simulink model "operativobuono"  (R2024a)
settings: Solver=VariableStepAuto  StartTime=0.0  StopTime=70  RelTol=1e-3
undefined symbols (not defined in the file or in its folder): DiscIntNeverNeededParam
settings Model: Creator=ThinkPad  LastModifiedBy=UTENTE
settings ModelReferenceCC: EnableRefExpFcnMdlSchedulingChecks=on
settings RTWCC: GPUComputeCapability=3.5

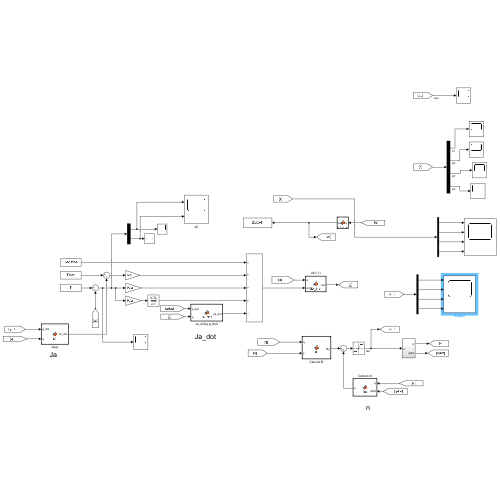
[thumbnail: Simulink's stored preview of the top-level diagram]
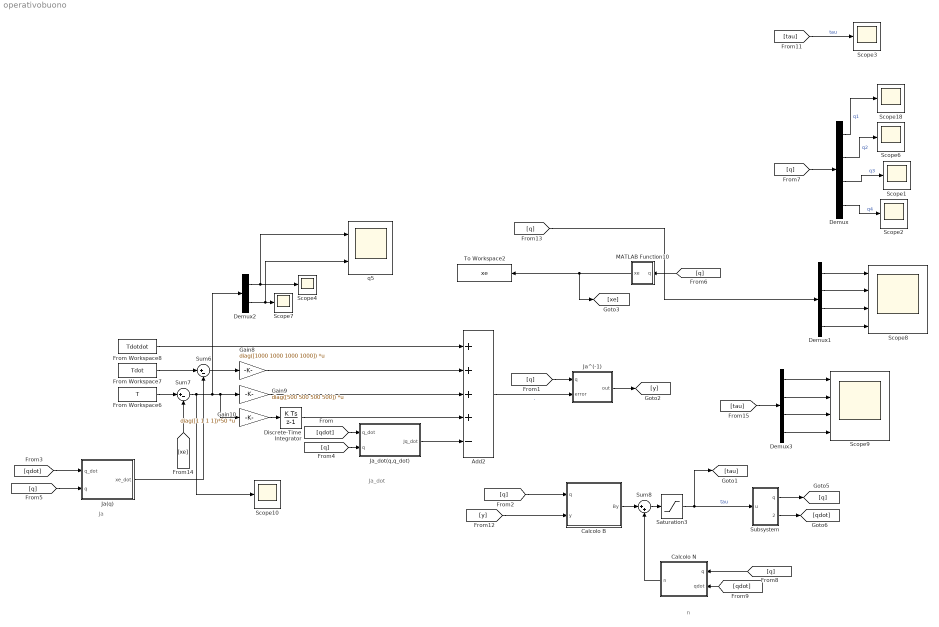
== system operativobuono ==
  note: n
  note: Ja
  note: Ja_dot
  Add2 : Sum  Inputs=++++-
  Calcolo B : MATLAB Function  TreatAsAtomicUnit=on
  Calcolo N : MATLAB Function  TreatAsAtomicUnit=on
  Demux : Demux
  Demux1 : Demux
  Demux2 : Demux  Outputs=[3 1]
  Demux3 : Demux
  Discrete-Time Integrator : DiscreteIntegrator  InitialCondition=[0 0 0 0]'  SampleTime=0.001  ICPrevOutput=DiscIntNeverNeededParam  ICPrevScaledInput=DiscIntNeverNeededParam
  From Workspace6 : FromWorkspace  VariableName=T  SampleTime=0.001
  From Workspace7 : FromWorkspace  VariableName=Tdot  SampleTime=0.001
  From Workspace8 : FromWorkspace  VariableName=Tdotdot
  Gain10 : Gain  Gain=diag([1 1 1 1])*50  Multiplication=Matrix(K*u)
  Gain8 : Gain  Gain=diag([1000 1000 1000 1000])  Multiplication=Matrix(K*u)
  Gain9 : Gain  Gain=diag([500 500 500 500])  Multiplication=Matrix(K*u)
  Ja(q) : MATLAB Function  TreatAsAtomicUnit=on
  Ja^(-1) : MATLAB Function  TreatAsAtomicUnit=on
  Ja_dot(q,q_dot) : MATLAB Function  TreatAsAtomicUnit=on
  MATLAB Function10 : MATLAB Function  TreatAsAtomicUnit=on
  Saturation3 : Saturate  UpperLimit=[1 1 1 1]*300  LowerLimit=-[1 1 1 1]*300
  Scope{1..4,6..7,10,18} (8 alike) : Scope
  Scope8 : Scope  NumInputPorts=4
  Scope9 : Scope  NumInputPorts=4
  Subsystem : Subsystem
  Sum6 : Sum  Inputs=|+-
  Sum7 : Sum  Inputs=|+-
  Sum8 : Sum  Inputs=|++
  To Workspace2 : ToWorkspace  VariableName=xe  SampleTime=0.001
  q5 : Scope  NumInputPorts=2
  wires:
  Ja(q)/1(xe_dot) -> Sum6/2
  Demux3/3 -> Scope9/3
  [q] -> MATLAB Function10/1(q)
  Calcolo N/1(n) -> Sum8/2
  [q] -> Demux/1
  Demux3/4 -> Scope9/4
  Gain9/1 -> Add2/3
  [qdot] -> Calcolo N/2(qdot)
  From Workspace8/1 -> Add2/1
  Demux1/2 -> Scope8/2
  Discrete-Time Integrator/1 -> Add2/4
  Demux1/4 -> Scope8/4
  Demux2/1 -> q5/1, Scope4/1
  Demux2/2 -> q5/2, Scope7/1
  Sum7/1 -> Scope10/1, Demux2/1, Gain9/1, Gain10/1
  [y] -> Calcolo B/2(y)
  [q] -> Ja(q)/2(q)
  Demux3/1 -> Scope9/1
  Sum6/1 -> Gain8/1
  Subsystem/1(q) -> [q]
  Sum8/1 -> Saturation3/1
  From Workspace7/1 -> Sum6/1
  From Workspace6/1 -> Sum7/1
  MATLAB Function10/1(xe) -> [xe], To Workspace2/1
  Add2/1 -> Ja^(-1)/2(error)  "."
  Gain10/1 -> Discrete-Time Integrator/1
  [qdot] -> Ja_dot(q,q_dot)/1(q_dot)
  Demux1/3 -> Scope8/3
  Demux1/1 -> Scope8/1
  Calcolo B/1(By) -> Sum8/1
  [q] -> Calcolo N/1(q)
  [q] -> Calcolo B/1(q)
  Gain8/1 -> Add2/2
  [tau] -> Scope3/1  "tau"
  Ja_dot(q,q_dot)/1(Jq_dot) -> Add2/5
  Demux/4 -> Scope2/1  "q4"
  [qdot] -> Ja(q)/1(q_dot)
  Demux3/2 -> Scope9/2
  [q] -> Ja_dot(q,q_dot)/2(q)
  Subsystem/2(qdot) -> [qdot]
  Saturation3/1 -> Subsystem/1(u), [tau]  "tau"
  Demux/2 -> Scope6/1  "q2"
  Ja^(-1)/1(out) -> [y]
  Demux/1 -> Scope18/1  "q1"
  [q] -> Ja^(-1)/1(q)
  Demux/3 -> Scope1/1  "q3"
  [q] -> Demux1/1
  [xe] -> Sum7/2
  [tau] -> Demux3/1

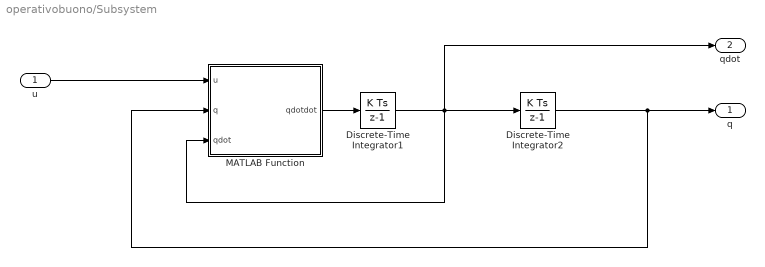
== system operativobuono/Subsystem ==
  u : Inport
  Discrete-Time Integrator1 : DiscreteIntegrator  InitialCondition=[0 0 0 0]'  SampleTime=0.001  ICPrevOutput=DiscIntNeverNeededParam  ICPrevScaledInput=DiscIntNeverNeededParam
  Discrete-Time Integrator2 : DiscreteIntegrator  InitialCondition=[pi/4,pi/6,pi/5,0.5]'  SampleTime=0.001  ICPrevOutput=DiscIntNeverNeededParam  ICPrevScaledInput=DiscIntNeverNeededParam
  MATLAB Function : MATLAB Function  TreatAsAtomicUnit=on
  q : Outport
  qdot : Outport  Port=2
  wires:
  MATLAB Function/1(qdotdot) -> Discrete-Time Integrator1/1
  Discrete-Time Integrator2/1 -> q/1, MATLAB Function/2(q)
  u/1 -> MATLAB Function/1(u)
  Discrete-Time Integrator1/1 -> qdot/1, MATLAB Function/3(qdot), Discrete-Time Integrator2/1

== matlab function operativobuono/Ja(q) ==
  data: q_dot input; q input; xe_dot output
function xe_dot = JA(q_dot, q)

J=[-0.5*sin(q(1))-0.5*sin(q(1)+q(2)) -0.5*sin(q(1)+q(2)) 0 0;
    0.5*cos(q(1))+0.5*cos(q(1)+q(2)) 0.5*cos(q(1)+q(2)) 0 0;
    0 0 -1 0;
    1 1 0 -1];
xe_dot=J*q_dot;
end

== matlab function operativobuono/Ja^(-1) ==
  data: q input; out output; error input
function out= JA_inv(q,error)

J=[-0.5*sin(q(1))-0.5*sin(q(1)+q(2)) -0.5*sin(q(1)+q(2)) 0 0;
    0.5*cos(q(1))+0.5*cos(q(1)+q(2)) 0.5*cos(q(1)+q(2)) 0 0;
    0 0 -1 0;
    1 1 0 -1];

J_inv=inv(J);

 inverse_Jacobian=J_inv;
 out = inverse_Jacobian*error;
end

== matlab function operativobuono/MATLAB Function10 ==
  data: q input; xe output
function xe = cinematica_diretta(q)
% T_4_0=[cos(q(4))*(cos(q(1))*cos(q(2))-sin(q1)*sin(q2))+sin(q(4))*(cos(q1)*sin(q(2))+cos(q(2))*sin(q(1)))   cos(q(4))*(cos(q(1))*sin(q(2))+cos(q(2))*sin(q(1)))-sin(q(4))*(cos(q(1))*cos(q(2))-sin(q(1))*sin(q(2)))  0 cos(q(1))/2+(cos(q(1))*cos(q(2)))/2-(sin(q(1))*sin(q(2)))/2;
%         cos(q(4))*(cos(q(1))*sin(q(2))+cos(q(2))*sin(q(1)))-sin(q(4))*(cos(q(1))*cos(q(2))-sin(q(1))*sin(q(2))) -cos(q(4))*(cos(q(1))*cos(q(2))-sin(q(1))*sin(q(2)))-sin(q(4))*(cos(q(1))*sin(q(2))+cos(q(2))*sin(q(1)))  0 sin(q(1))/2+(cos(q(1))*sin(q(2)))/2+(cos(q(2))*sin(q(2)))/2;
%                       0                                                      0                    -1                                                1-q(3);
%         0                                       0                                         0                                                                                                                                      1];

x_e=[0.5*cos(q(1))+0.5*cos(q(1)+q(2));
    0.5*sin(q(1))+0.5*sin(q(1)+q(2));
        1-q(3);
        q(1)+q(2)-q(4)];
xe=x_e;
end

== matlab function operativobuono/Calcolo N ==
  data: n output; q input; qdot input
function n = fcn(q, qdot)
d0=1;
a1=0.5;
a2=0.5;
l1=0.25;
l2=0.25;
ml1=20;
ml2=20;
ml3=10;
Il1=4;
Il2=4;
Il4=1;
kr1=1;
kr2=1;
kr3=50;
kr4=20;
Im1=0,01;
Im2=0,01;
Im3=0,005;
Im4=0,001;
Fm1=0.00005;
Fm2=0.00005;
Fm3=0.01;
Fm4=0.005;
ml=3;
mm1=0;
mm2=0;
mm3=0;
mm4=0;

Jp_l1=[-l1*sin(q(1)) 0 0  0;
        l1*cos(q(1)) 0 0  0;
        0            0 0  0];
    
Jo_l1=[0 0 0 0;
       0 0 0 0;
       1 0 0 0];
   
Jp_l2=[-a1*sin(q(1))-l2*sin(q(1)+q(2)) -l2*sin(q(1)+q(2)) 0  0;
        a1*cos(q(1))+l2*cos(q(1)+q(2)) +l2*cos(q(1)+q(2)) 0  0;
        0                                      0          0  0];
   
Jo_l2=[0 0 0 0;
       0 0 0 0;
       1 1 0 0];

Jp_l3=[-a1*sin(q(1))-a2*sin(q(1)+q(2)) -a2*sin(q(1)+q(2))  0   0;
        a1*cos(q(1))+a2*cos(q(1)+q(2)) +a2*cos(q(1)+q(2))  0   0;
        0                                               0  -1  0];
Jo_l3=[0 0 0 0;
       0 0 0 0;
       1 1 0 0];
 
Jp_l4=[-a1*sin(q(1))-a2*sin(q(1)+q(2)) -a2*sin(q(1)+q(2))  0   0;
        a1*cos(q(1))+a2*cos(q(1)+q(2)) +a2*cos(q(1)+q(2))  0   0;
        0                                               0  -1  0];
Jo_l4=[0 0 0 0;
       0 0 0 0;
       1 1 0 -1];

Jp_m1=[0 0 0 0;
       0 0 0 0;
       0 0 0 0];
   
Jo_m1=[0 0 0 0;
       0 0 0 0;
       kr1 0 0 0];

Jp_m2=[-a1*sin(q(1)) 0 0 0;
       a1*cos(q(1)) 0 0 0;
           0        0 0 0];
       
Jo_m2=[0 0 0 0;
       0 0 0 0;
       1 kr2 0 0];

Jp_m3=[-a1*sin(q(1))-a2*sin(q(1)+q(2)) -a2*sin(q(1)+q(2))  0 0;
        a1*cos(q(1))+a2*cos(q(1)+q(2)) +a2*cos(q(1)+q(2))  0 0;
                      0                         0          0 0];

Jo_m3=[0 0 0 0;
       0 0 0 0;
       1 1 -kr3 0];

Jp_m4=[-a1*sin(q(1))-a2*sin(q(1)+q(2)) -a2*sin(q(1)+q(2))  0 0;
        a1*cos(q(1))+a2*cos(q(1)+q(2)) +a2*cos(q(1)+q(2))  0 0;
                      0                         0          -1 0];
Jo_m4=[0 0 0 0;
       0 0 0 0;
       1 1 0 -kr4];


Fv=diag([kr1^2*Fm1 kr2^2*Fm2 kr3^2*Fm3 kr4^2*Fm4]);
% Fv=[Fm1 0   0   0;
%     0   Fm2 0   0;
%     0   0   Fm3 0;
%     0   0   0   Fm4];

g=[0 0 -9.81*(ml3) 0]';

Jpl1_dq1=[-l1*cos(q(1)) 0 0 0;
    -l1*sin(q(1)) 0 0 0;
    0 0 0 0];

Jpl2_dq1=[-a1*cos(q(1))-l2*cos(q(1)+q(2)) -l2*cos(q(1)+q(2)) 0 0;
    -a1*sin(q(1))-l2*sin(q(1)+q(2)) -l2*sin(q(1)+q(2)) 0 0;
    0 0 0 0];

Jpl2_dq2=[-a2*cos(q(1)+q(2)) -a2*cos(q(1)+q(2)) 0 0;
    -a2*sin(q(1)+q(2)) -a2*sin(q(1)+q(2)) 0 0;
    0 0 0 0];

Jpl4_dq1=[-a1*cos(q(1))-a2*cos(q(1)+q(2)) -a2*cos(q(1)+q(2)) 0 0;
    -a1*sin(q(1))-a2*sin(q(1)+q(2)) -a2*sin(q(1)+q(2)) 0 0;
    0 0 0 0];

Jpl4_dq2=[-a2*sin(q(1)+q(2)) -a2*sin(q(1)+q(2)) 0 0;
    -a2*cos(q(1)+q(2)) -a2*cos(q(1)+q(2)) 0 0;
    0 0 0 0];

dBdq1=ml1*(Jpl1_dq1'*Jp_l1+Jp_l1'*Jpl1_dq1)+ml2*(Jpl2_dq1'*Jp_l2+Jp_l2'*Jpl2_dq1)...
    +ml3*(Jpl4_dq1'*Jp_l4+Jp_l4'*Jpl4_dq1);

dBdq2=ml2*(Jpl2_dq2'*Jp_l2+Jp_l2'*Jpl2_dq2)+ml3*(Jpl4_dq2'*Jp_l4+Jp_l4'*Jpl4_dq2);

H=zeros(4,4,4);


for i=1:4
    for j=1:4
        for k=1:4
            H(i,j,k)=0;
        end
    end
end

H(1,1,2)=1/2*(dBdq2(1,1)+dBdq1(1,2)-dBdq1(1,2));
H(1,2,1)=H(1,1,2); 
H(1,2,2)=1/2*(dBdq2(1,2)+dBdq2(1,2)-dBdq1(2,2));
H(2,1,1)=1/2*(dBdq1(2,1)+dBdq1(2,1)-dBdq2(1,1));
H(2,1,2)=1/2*(dBdq2(2,1)+dBdq1(2,2)-dBdq2(1,2));
H(2,2,1)=H(2,1,2);
H(2,2,2)=1/2*(dBdq2(2,2)+dBdq2(2,2)-dBdq2(2,2));

C=zeros(4,4);
for i=1:4
    for j=1:4
        C(i,j)=0;
    end
end

for i=1:4
    for j=1:4
        for k=1:4
            r=H(i,j,k)*qdot(k);
            C(i,j)=C(i,j)+r;
        end
    end
end

n=C*qdot+Fv*qdot+g;

end

== matlab function operativobuono/Ja_dot(q,q_dot) ==
  data: q_dot input; q input; Jq_dot output
function Jq_dot = JA_dot(q_dot, q)
J_dot=[-0.5*cos(q(1))*q_dot(1)-0.5*cos(q(1)+q(2))*(q_dot(1)+q_dot(2)) -0.5*cos(q(1)+q(2))*(q_dot(1)+q_dot(2)) 0 0;
    -0.5*sin(q(1))*q_dot(1)-0.5*sin(q(1)+q(2))*(q_dot(1)+q_dot(2)) -0.5*sin(q(1)+q(2))*(q_dot(1)+q_dot(2)) 0 0;
    0 0 0 0;
    0 0 0 0];
Jq_dot=J_dot*q_dot;
end

== matlab function operativobuono/Calcolo B ==
  data: q input; y input; By output
function By = B(q, y)
    d0=1; 
    a1=0.5; 
    a2=0.5; 
    l1=0.25; 
    l2=0.25; 
    ml1=20; 
    ml2=20; 
    ml3=10; 
    ml4=0; 
    Il1=4; 
    Il2=4; 
    Il3=0;
    Il4=1; 
    Kr1=1;
    Kr2=1;
    Kr3=50; 
    Kr4 =20;
    Im1=0.01; 
    Im2=0.01; 
    Im3=0.005; 
    Im4=0.001;
    Fm1=0.00005; 
    Fm2=0.00005; 
    Fm3=0.01; 
    Fm4 =0.005; 
    mm1=0;
    mm2=0;
    mm3=0;
    mm4=0;
    ml=3;
    
    Jp_l1=[-l1*sin(q(1)) 0 0 0; 
            l1*cos(q(1)) 0 0 0; 
            0 0 0 0];
    Jo_l1=[zeros(2,4)
           1 0 0 0];
    
    Jp_l2=[-a1*sin(q(1))-l2*sin(q(1)+q(2)) -l2*sin(q(1)+q(2)) 0 0; 
            a1*cos(q(1))+l2*cos(q(1)+q(2)) l2*cos(q(1)+q(2)) 0 0;
            0 0 0 0];
    Jo_l2=[zeros(2,4)
           1 1 0 0];
    
    Jp_l3=[-a1*sin(q(1))-a2*sin(q(1)+q(2)) -a2*sin(q(1)+q(2)) 0 0; 
            a1*cos(q(1))+a2*cos(q(1)+q(2)) a2*cos(q(1)+q(2)) 0 0;
            0 0 -1 0];
    Jo_l3 = [zeros(2,4)
             1 1 0 0];
    
    Jp_l4=Jp_l3;
    Jo_l4 = [zeros(2,4)
             1 1 0 -1];
    
    Jp_m1 = [0 0 0 0;
             0 0 0 0;
             0 0 0 0];
    Jo_m1 = [zeros(2,4)
             Kr1 0 0 0];
    
    Jp_m2 = [-a1*sin(q(1)) 0 0 0; 
            a1*cos(q(1)) 0 0 0; 
            0 0 0 0];
    Jo_m2 = [zeros(2,4)
             1 Kr2 0 0];
    
    Jp_m3 = [-a1*sin(q(1))-a2*sin(q(1)+q(2)) -a2*sin(q(1)+q(2)) 0 0; 
              a1*cos(q(1))+a2*cos(q(1)+q(2)) a2*cos(q(1)+q(2)) 0 0;
              0 0 0 0];
    Jo_m3 = [zeros(2,4)
             1 1 -Kr3 0];
    
    Jp_m4 = [-a1*sin(q(1))-a2*sin(q(1)+q(2)) -a2*sin(q(1)+q(2)) 0 0; 
              a1*cos(q(1))+a2*cos(q(1)+q(2)) a2*cos(q(1)+q(2)) 0 0;
              0 0 -1 0];
    Jo_m4 = [zeros(2,4)
             1 1 0 -Kr4];
    B1 = ml1*Jp_l1'*Jp_l1+Jo_l1'*Il1*Jo_l1+mm1*Jp_m1'*Jp_m1+Jo_m1'*Im1*Jo_m1;
    B2 = ml2*Jp_l2'*Jp_l2+Jo_l2'*Il2*Jo_l2+mm2*Jp_m2'*Jp_m2+Jo_m2'*Im2*Jo_m2;
    B3 = ml3*Jp_l3'*Jp_l3+Jo_l3'*Il3*Jo_l3+mm3*Jp_m3'*Jp_m3+Jo_m3'*Im3*Jo_m3;
    B4 = (ml4)*Jp_l4'*Jp_l4+Jo_l4'*Il4*Jo_l4+mm4*Jp_m4'*Jp_m4+Jo_m4'*Im4*Jo_m4;
    B = B1+B2+B3+B4;
    
    By=B*y;

end

== matlab function operativobuono/Subsystem/MATLAB Function ==
  data: u input; q input; qdot input; qdotdot output
function qdotdot = fcn(u, q, qdot)
    d0=1; %m
    a1=0.5; %m
    a2=0.5; %m
    
    l1=0.25; %m
    l2=0.25; %m
    ml1=20; %kg
    ml2=20; %kg
    ml3=10; %kg
    ml4=0; %kg
    Il1=4; %kg�m2
    Il2=4; %kg�m2
    Il3=0;
    Il4=1; %kg�m2
    Kr1=1;
    Kr2=1;
    Kr3=50; %rad/m
    Kr4 =20;
    Im1=0.01; %kg�m2
    Im2=0.01; %kg�m2
    Im3=0.005; %kg�m2
    Im4=0.001;%kg
    Fm1=0.00005; %N�m�s/rad
    Fm2=0.00005; %N�m�s/rad
    Fm3=0.01; %N�m�s/rad
    Fm4 =0.005; %N�m�s/rad
    mm1=0;
    mm2=0;
    mm3=0;
    mm4=0;
    ml=3;
    
    Jp_l1=[-l1*sin(q(1)) 0 0 0; 
            l1*cos(q(1)) 0 0 0; 
            0 0 0 0];
    Jo_l1=[zeros(2,4)
           1 0 0 0];
    
    Jp_l2=[-a1*sin(q(1))-l2*sin(q(1)+q(2)) -l2*sin(q(1)+q(2)) 0 0; 
            a1*cos(q(1))+l2*cos(q(1)+q(2)) l2*cos(q(1)+q(2)) 0 0;
            0 0 0 0];
    Jo_l2=[zeros(2,4)
           1 1 0 0];
    
    Jp_l3=[-a1*sin(q(1))-a2*sin(q(1)+q(2)) -a2*sin(q(1)+q(2)) 0 0; 
            a1*cos(q(1))+a2*cos(q(1)+q(2)) a2*cos(q(1)+q(2)) 0 0;
            0 0 -1 0];
    Jo_l3 = [zeros(2,4)
             1 1 0 0];
    
    Jp_l4=Jp_l3;
    Jo_l4 = [zeros(2,4)
             1 1 0 -1];
    
    Jp_m1 = [0 0 0 0;
             0 0 0 0;
             0 0 0 0];
    Jo_m1 = [zeros(2,4)
             Kr1 0 0 0];
    
    Jp_m2 = [-a1*sin(q(1)) 0 0 0; 
            a1*cos(q(1)) 0 0 0; 
            0 0 0 0];
    Jo_m2 = [zeros(2,4)
             1 Kr2 0 0];
    
    Jp_m3 = [-a1*sin(q(1))-a2*sin(q(1)+q(2)) -a2*sin(q(1)+q(2)) 0 0; 
              a1*cos(q(1))+a2*cos(q(1)+q(2)) a2*cos(q(1)+q(2)) 0 0;
              0 0 0 0];
    Jo_m3 = [zeros(2,4)
             1 1 -Kr3 0];
    
    Jp_m4 = [-a1*sin(q(1))-a2*sin(q(1)+q(2)) -a2*sin(q(1)+q(2)) 0 0; 
              a1*cos(q(1))+a2*cos(q(1)+q(2)) a2*cos(q(1)+q(2)) 0 0;
              0 0 -1 0];
    Jo_m4 = [zeros(2,4)
             1 1 0 -Kr4];
    B1 = ml1*Jp_l1'*Jp_l1+Jo_l1'*Il1*Jo_l1+mm1*Jp_m1'*Jp_m1+Jo_m1'*Im1*Jo_m1;
    B2 = ml2*Jp_l2'*Jp_l2+Jo_l2'*Il2*Jo_l2+mm2*Jp_m2'*Jp_m2+Jo_m2'*Im2*Jo_m2;
    B3 = ml3*Jp_l3'*Jp_l3+Jo_l3'*Il3*Jo_l3+mm3*Jp_m3'*Jp_m3+Jo_m3'*Im3*Jo_m3;
    B4 = (ml4+ml)*Jp_l4'*Jp_l4+Jo_l4'*Il4*Jo_l4+mm4*Jp_m4'*Jp_m4+Jo_m4'*Im4*Jo_m4;
    B = B1+B2+B3+B4;
    
    Fv = diag([Kr1^2*Fm1 Kr2^2*Fm2 Kr3^2*Fm3 Kr4^2*Fm4]);
    g=[0 0 -9.81*(ml+ml3) 0]';
    
Jpl1_dq1=[-l1*cos(q(1)) 0 0 0;
    -l1*sin(q(1)) 0 0 0;
    0 0 0 0];

Jpl2_dq1=[-a1*cos(q(1))-l2*cos(q(1)+q(2)) -l2*cos(q(1)+q(2)) 0 0;
    -a1*sin(q(1))-l2*sin(q(1)+q(2)) -l2*sin(q(1)+q(2)) 0 0;
    0 0 0 0];

Jpl2_dq2=[-a2*cos(q(1)+q(2)) -a2*cos(q(1)+q(2)) 0 0;
    -a2*sin(q(1)+q(2)) -a2*sin(q(1)+q(2)) 0 0;
    0 0 0 0];

Jpl4_dq1=[-a1*cos(q(1))-a2*cos(q(1)+q(2)) -a2*cos(q(1)+q(2)) 0 0;
    -a1*sin(q(1))-a2*sin(q(1)+q(2)) -a2*sin(q(1)+q(2)) 0 0;
    0 0 0 0];

Jpl4_dq2=[-a2*sin(q(1)+q(2)) -a2*sin(q(1)+q(2)) 0 0;
    -a2*cos(q(1)+q(2)) -a2*cos(q(1)+q(2)) 0 0;
    0 0 0 0];

% Calcolo matrice differenziate rispetto a dq1 dq2
dBdq1=ml1*(Jpl1_dq1'*Jp_l1+Jp_l1'*Jpl1_dq1)+ml2*(Jpl2_dq1'*Jp_l2+Jp_l2'*Jpl2_dq1)...
    +ml3*(Jpl4_dq1'*Jp_l4+Jp_l4'*Jpl4_dq1);

dBdq2=ml2*(Jpl2_dq2'*Jp_l2+Jp_l2'*Jpl2_dq2)+ml3*(Jpl4_dq2'*Jp_l4+Jp_l4'*Jpl4_dq2);

H=zeros(4,4,4);

% Inizializzazione simboli cristoffel del primo tipo
for i=1:4
    for j=1:4
        for k=1:4
            H(i,j,k)=0;
        end
    end
end

H(1,1,2)=1/2*(dBdq2(1,1)+dBdq1(1,2)-dBdq1(1,2));
H(1,2,1)=H(1,1,2); 
H(1,2,2)=1/2*(dBdq2(1,2)+dBdq2(1,2)-dBdq1(2,2));
H(2,1,1)=1/2*(dBdq1(2,1)+dBdq1(2,1)-dBdq2(1,1));
H(2,1,2)=1/2*(dBdq2(2,1)+dBdq1(2,2)-dBdq2(1,2));
H(2,2,1)=H(2,1,2);
H(2,2,2)=1/2*(dBdq2(2,2)+dBdq2(2,2)-dBdq2(2,2));


% C=sym('C',[4,4]);
C=zeros(4,4);
for i=1:4
    for j=1:4
        C(i,j)=0;
    end
end

% qdot=sym('qdot',[4,1]);

for i=1:4
    for j=1:4
        for k=1:4
            r=H(i,j,k)*qdot(k);
            C(i,j)=C(i,j)+r;
        end
    end
end
    
qdotdot = inv(B)*(u-C*qdot-Fv*qdot-g);
end
